simulink model "testemplannerglf_cs"  (R2020a)
settings: Solver=ode5  StartTime=0.0  StopTime=75  FixedStep=1/1000  RelTol=1e-3
PreLoadFcn:
  | mbxruntime.callbacks.PreLoadFcn(bdroot);
PostLoadFcn:
  | mbxruntime.callbacks.PostLoadFcn(bdroot);
InitFcn:
  | mbxruntime.callbacks.InitFcn(bdroot);
StartFcn:
  | mbxruntime.callbacks.StartFcn(bdroot);
StopFcn:
  | mbxruntime.callbacks.StopFcn(bdroot);
model workspace (MAT data in the model file):
  mbox_table : object (value not decoded)
  model_closed = 0
  sim_status = 0
values from neighbouring files (symbols this model uses):
  global_path_x = [-3.342 -2.8421723782 -2.34265574205 -1.8434543045 -1.34457058078 -0.846006057582 -0.347761597731 0.15016231435 0.647765423738 1.14504761469 1.64200885585 2.13864916705 ... (1501 elements, 1501x1)]    [global_path.mat]
  global_path_y = [4.7606 4.76495870158 4.76931469124 4.77366793224 4.77801840264 4.78236608949 4.78671098525 4.7910530857 4.79539238863 4.79972889301 4.80406259858 4.80839350551 ... (1501 elements, 1501x1)]    [global_path.mat]
undefined symbols (not defined in the file or in its folder): DiscIntNeverNeededParam, warningInitialVelocity, x0
libraries: simulink x19, PreScanSimulinkLibrary x11, simulink_extras x6, Solver_SF x1
(part 7 of 7)

== matlab function testemplannerglf_cs/Audi_A8_Sedan_1/decesion&&planning/referenceline provider/project_point ==
  data: host_x input; match_point_index_set output; host_y input; frenet_x input; frenet_y input; frenet_heading input; frenet_kappa input; project_x_set output; project_y_set output; project_heading_set output; project_kappa_set output
function [match_point_index_set,project_x_set,project_y_set,project_heading_set,project_kappa_set] =...
    fcn(host_x,host_y,frenet_x,frenet_y,frenet_heading,frenet_kappa)
%功能：该函数是为了求投影点的x，y,heading,kappa值，其中分成了首次运行和非首次运行，非首次运行条件下可以利用上一个周期运行的结果加速运算
%输入：host_x,host_y,frenet_x,frenet_y,frenet_heading,frenet_kappa
%输出：match_point_index_set, project_x、y_set， project_heading_set,proj_kappa_set
%2022 0309 glf写于国实507

%输出初始化
n = 128;%128只是用来存储数据的，实际中只用了第一个点.之后可以试试如果n=1看看程序能不能运行！！！！！
match_point_index_set = ones(n,1) * nan;
project_x_set = ones(n,1) * nan;
project_y_set = ones(n,1) * nan;
project_heading_set = ones(n,1) * nan;
project_kappa_set = ones(n,1) * nan;

%声明持久变量
persistent isFirstRun;
persistent pre_match_point_index_set;
persistent pre_frenet_x_set;
persistent pre_frenet_y_set;
persistent pre_frenet_heading_set;
persistent pre_frenet_kappa_set;

if isempty(isFirstRun)
    isFirstRun = 0;
    pre_frenet_x_set = frenet_x;
    pre_frenet_y_set = frenet_y;
    pre_frenet_heading_set = frenet_heading;
    pre_frenet_kappa_set = frenet_kappa;
    %初始化match_point的结果
    pre_match_point_index_set = ones(n,1)*nan;
    
    for i = 1:length(host_x)
        if isnan(host_x(i))
           break; 
        end
        start_index = 1;
        min_distance = inf;
        increase_count = 0;
        for j = start_index:length(frenet_x)
            distance = sqrt((host_x(i) - frenet_x(j))^2 + (host_y(i) - frenet_y(j))^2);
            if distance < min_distance
               distance = min_distance;
               match_point_index_set(i) = j;
            else
                increase_count = increase_count + 1;
            end
            if increase_count == 50
               break; 
            end
        end
        
        %由匹配点求投影点
        match_point_index = match_point_index_set(i);
        match_point_index_x = pre_frenet_x_set(match_point_index);%这里源代码写的是frenet_path_x
        match_point_index_y = pre_frenet_y_set(match_point_index);
        %匹配点位失
        match_point_direction = [match_point_index_x;match_point_index_y];
        %带投影点位失
        host_direction = [host_x;host_y];
        match_point_index_heading = pre_frenet_heading_set(match_point_index);
        match_point_index_kappa = pre_frenet_kappa_set(match_point_index);
        ds = (host_direction - match_point_direction)'*[cos(match_point_index_heading);sin(match_point_index_heading)];
        proj_index_set = match_point_direction + ds*[cos(match_point_index_heading);sin(match_point_index_heading)];
        proj_index_heading = match_point_index_heading + ds * match_point_index_kappa;
        proj_index_kappa = match_point_index_kappa;
        
        %输出计算结果
        project_x_set(i) = proj_index_set(1);
        project_y_set(i) = proj_index_set(2);
        project_heading_set(i) = proj_index_heading;
        project_kappa_set(i) = proj_index_kappa;   
    end
    pre_match_point_index_set = match_point_index_set;
    
else
    for i = 1:length(host_x)
        
        start_index = pre_match_point_index_set(i);
        %以下判断语句是为了防止感知时出现bug，具体还不懂
        %声明increase_count_limit
        increase_count_limit = 5;
        if isnan(start_search_index)
            increase_count_limit = 50;
            %搜索起点设为1
            start_search_index = 1;            
        end
        increase_count = 0; 
        
        %由上一个匹配点计算车辆的行驶方向
        %匹配点位失
        vector_match_point_index = [pre_frenet_x_set(start_index);pre_frenet_y_set(start_index)];
        %待投影点位失
        vector_host_point_index = [host_x;host_y];
        match_point_index_heading = pre_frenet_heading_set(start_index);
        flag = (vector_host_point_index - vector_match_point_index)'*[cos(match_point_index_heading);sin(match_point_index_heading)];
        if flag > 0.001
            min_distance = inf;
            for j = start_index:length(frenet_x)
                distance = sqrt((host_x(i) - frenet_x(j))^2 + (host_y(i) - frenet_y(j))^2);
                if distance < min_distance
                   distance = min_distance;
                   match_point_index_set(i) = j;
                else
                    increase_count = increase_count + 1;
                end
                if increase_count == increase_count_limit
                   break; 
                end
            end
        elseif flag < -0.001
            min_distance = inf;
            for j = start_index:-1:1
                distance = sqrt((host_x(i) - frenet_x(j))^2 + (host_y(i) - frenet_y(j))^2);
                if distance < min_distance
                   distance = min_distance;
                   match_point_index_set(i) = j;
                else
                    increase_count = increase_count + 1;
                end
                if increase_count == increase_count_limit
                   break; 
                end
            end
        else
            match_point_index_set(i) = start_index;
        end
        
        %由匹配点求投影点
        match_point_index = match_point_index_set(i);
        match_point_index_x = pre_frenet_x_set(match_point_index);%这里源代码写的是frenet_path_x
        match_point_index_y = pre_frenet_y_set(match_point_index);
        %匹配点位失
        match_point_direction = [match_point_index_x;match_point_index_y];
        %带投影点位失
        host_direction = [host_x;host_y];
        match_point_index_heading = pre_frenet_heading_set(match_point_index);
        match_point_index_kappa = pre_frenet_kappa_set(match_point_index);
        ds = (host_direction - match_point_direction)'*[cos(match_point_index_heading);sin(match_point_index_heading)];
        proj_index_set = match_point_direction + ds*[cos(match_point_index_heading);sin(match_point_index_heading)];
        proj_index_heading = match_point_index_heading + ds * match_point_index_kappa;
        proj_index_kappa = match_point_index_kappa;
        
        %输出计算结果
        project_x_set(i) = proj_index_set(1);
        project_y_set(i) = proj_index_set(2);
        project_heading_set(i) = proj_index_heading;
        project_kappa_set(i) = proj_index_kappa; 
    end
    pre_frenet_x_set = frenet_x;
    pre_frenet_y_set = frenet_y;
    pre_frenet_heading_set = frenet_heading;
    pre_frenet_kappa_set = frenet_kappa;
    pre_match_point_index_set = match_point_index_set;
end

== matlab function testemplannerglf_cs/Audi_A8_Sedan_2/PathFollower_Preview_1/LateralController/CTRL REFERENCES/Calculate Lateral Error/eml_find_10k_lateral_error_points ==
  data: pvp input size=2; dist_psvehicle output size=10; TrajOffset_x_y_Y input size=3; ActorOffset_Left_Right input; p0 input size=2; PreviewDistance input size=10; Traj_x parameter; Traj_y parameter; Traj_t parameter; Traj_v parameter; RefreshCounter parameter
function dist_psvehicle  = eml_find_10k_lateral_error_points(pvp,TrajOffset_x_y_Y,ActorOffset_Left_Right,p0,PreviewDistance,Traj_x,Traj_y,Traj_t,Traj_v,RefreshCounter)

dist_psvehicle = emlfcn_find_10k_lateral_error_points(pvp,TrajOffset_x_y_Y,ActorOffset_Left_Right,p0,PreviewDistance,Traj_x,Traj_y,Traj_t,Traj_v,RefreshCounter);

% end function

== matlab function testemplannerglf_cs/Audi_A8_Sedan_1/decesion&&planning/referenceline provider/calc_heading_kappa ==
  data: path_x input; frenet_heading output; path_y input; frenet_kappa output
function [frenet_heading,frenet_kappa] = fcn(path_x,path_y)
%功能：该函数是利用已知的路径点计算heading和Kappa的值
%输入：path_x，path_y，全局路径点
%输出：frenet_heading，kappa
%2022 0310 glf 于寝室302

%注意事项，这里要注意角度的多值性，
%计算kappa时，kappa = dheading/ds，如果dheading差pi时tan值相等
%x和x+2pi往往代表同一个角度，但是（0.1-（-0.1））/ds和（0.1-（-0.1+2*pi））/ds差距较大
dx = diff(path_x);
dy = diff(path_y);

dx_pre = [dx(1);dx];
dx_after = [dx;dx(end)];
dx_final = (dx_pre + dx_after) / 2;

dy_pre = [dy(1);dy];
dy_after = [dy;dy(end)];
dy_final = (dy_pre + dy_after) / 2;

frenet_heading = atan2(dy_final,dx_final);

ds = sqrt(dx_final.^2 + dy_final.^2);
dheading = diff(frenet_heading);
dheading_pre = [dheading(1);dheading];
dheading_after = [dheading;dheading(end)];
dheading_final = (dheading_pre + dheading_after) / 2;

%为了防止dheading出现多了一个2pi的错误，假设真实的dheading较小，用sin（dheading）近似dheading
frenet_kappa = sin(dheading_final). / ds;

== matlab function testemplannerglf_cs/Audi_A8_Sedan_2/PathFollower_Preview_1/LateralController/CTRL REFERENCES/Find Reference Point (pref0) on Trajectory closest to P0 Point (p0)/eml_find_closest_trajectory_points0 ==
  data: pvp input size=2; Actor_traj_distance output; TrajOffset_x_y_Y input size=3; ActorOffset_Left_Right input; p0 input size=3; Traj_x parameter; Traj_y parameter; Actor_traj_angle output; RefreshCounter parameter
function [Actor_traj_distance,Actor_traj_angle]  = eml_find_closest_trajectory_points0(pvp,TrajOffset_x_y_Y,ActorOffset_Left_Right,p0,Traj_x,Traj_y,RefreshCounter)

[Actor_traj_distance,Actor_traj_angle]  = emlfcn_find_closest_trajectory_points0(pvp,TrajOffset_x_y_Y,ActorOffset_Left_Right,p0,Traj_x,Traj_y,RefreshCounter);

% end function

== matlab function testemplannerglf_cs/Audi_A8_Sedan_1/decesion&&planning/referenceline provider/180 ==
  data: match_point_index input; referenceline_x_set output; global_path_x input; global_path_y input; referenceline_y_set output
function [referenceline_x_set,referenceline_y_set] = fcn(match_point_index,global_path_x,global_path_y)
%功能：该函数是为了求参考线上180个点的坐标，一共选取181个点，从匹配点开始往前取150个点，往后取30个点，加上匹配点一共是181个点
%输入：match_point_index_set是匹配点的索引
%global_path_x、y:全局路径
%输出：referenceline_x、y_set参考线上的所有点

start_index = -1;
if match_point_index - 30 < 1%匹配点太靠前了
    start_index = 1;
elseif match_point_index + 150 > length(global_path_x) %匹配点太靠后了
    start_index = length(global_path_x) - 180;
else
    start_index = match_point_index;
end
%提取路径
referenceline_x_set = global_path_x(start_index:start_index + 180);
referenceline_y_set = global_path_y(start_index:start_index + 180);
